simulink model "FormulaElectric"  (R2015a)
settings: Solver=ode1  StartTime=0.0  StopTime=inf  FixedStep=0.001  RelTol=1e-3
InitFcn:
  | %init_dyn_platform
  | FEParameters
StartFcn:
  | tic
StopFcn:
  | toc
undefined symbols (not defined in the file): Battery, Env, magnitude, Motor, RPM2Rad
libraries: vehicleLib x22, mblibv1 x15, driveline x12, fl_lib x8, simulink x6, AMKMotor x4, nesl_utility x4, WheelAssembly x4, ephysenetlib x2, ControllerLib x1, simulink_extras x1
(part 1 of 4)
settings Model: SimulationMode=accelerator  CovSFcnEnable=off  ExtModeTrigDuration=100  Creator=Administrator  LastModifiedBy=tbria
settings SolverCC: ExtrapolationOrder=1
settings DataIOCC: LimitDataPoints=off  MaxDataPoints=1e6  SaveFinalState=on  SaveFormat=StructureWithTime  SaveOutput=off  SaveState=on  SignalLogging=off  StateSaveName=tmp_raccel_xout  SignalLoggingName=tmp_raccel_logsout
settings OptimizationCC: ExpressionDepthLimit=2147483647  InitFltsAndDblsToZero=on  EfficientMapNaN2IntZero=off  SimCompilerOptimization=on
settings DebuggingCC: UnderspecifiedInitializationDetection=Classic  MergeDetectMultiDrivingBlocksExec=none  SolverPrmCheckMsg=warning  InheritedTsInSrcMsg=none  MultiTaskDSMMsg=warning  MultiTaskCondExecSysMsg=none  Int32ToFloatConvMsg=none  ParameterPrecisionLossMsg=none  FcnCallInpInsideContextMsg=EnableAllAsWarning  StateNameClashWarn=warning
settings HardwareCC: ProdHWDeviceType=Generic->32-bit Real-Time Simulator  TargetLongLongMode=on  TargetIntDivRoundTo=Zero  TargetEndianess=LittleEndian  TargetHWDeviceType=MATLAB Host  ProdEqTarget=off
settings CodeAppCC: MaxIdLength=128
settings GRTTargetCC: CombineOutputUpdateFcns=off  GRTInterface=on
settings SimscapeCC: SelectedTab=Simscape

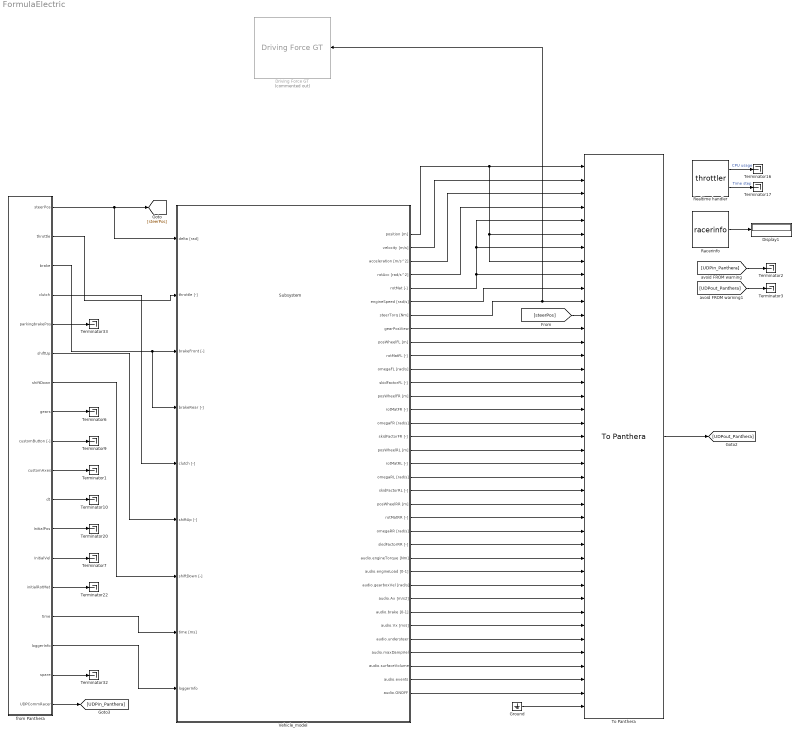
== system FormulaElectric ==
  Display1 : Display
  Driving Force GT : ControllerLib/Driving Force GT  Commented=on
  Ground : Ground
  Racerinfo : S-Function  Priority=5  FunctionName=racerinfo  Parameters=3
  Realtime handler : S-Function  FunctionName=throttler  Parameters=1
  Subsystem : Subsystem
      mask Display: image(imread('crudenlogo_small.jpg','jpg'))
  Terminator{1..3,6..7,9..10,16..17,20,22,32..33} (13 alike) : Terminator
  To Panthera : ephysenetlib/Output blocks/To Panthera
  Vehicle_model : Subsystem
  from Panthera : Subsystem
  wires:
  Vehicle_model/11(omegaFL [rad/s]) -> To Panthera/16
  Vehicle_model/13(posWheelFR [m]) -> To Panthera/18
  Vehicle_model/23(omegaRR [rad/s]) -> To Panthera/28
  To Panthera/1 -> [UDPout_Panthera]
  Vehicle_model/2(velocity [m/s]) -> To Panthera/2
  Vehicle_model/3(acceleration [m/s^2]) -> To Panthera/3
  Vehicle_model/8(gearPosView) -> To Panthera/13
  Vehicle_model/10(rotMatFL [-]) -> To Panthera/15
  Vehicle_model/14(rotMatFR [-]) -> To Panthera/19
  Vehicle_model/12(skidFactorFL [-]) -> To Panthera/17
  Vehicle_model/16(skidFactorFR [-]) -> To Panthera/21
  Vehicle_model/21(posWheelRR [m]) -> To Panthera/26
  Vehicle_model/18(rotMatRL [-]) -> To Panthera/23
  Vehicle_model/22(rotMatRR [-]) -> To Panthera/27
  Vehicle_model/19(omegaRL [rad/s]) -> To Panthera/24
  Vehicle_model/20(skidFactorRL [-]) -> To Panthera/25
  Vehicle_model/24(skidFactorRR [-]) -> To Panthera/29
  Vehicle_model/4(rotAcc [rad/s^2]) -> To Panthera/4
  Vehicle_model/15(omegaFR [rad/s]) -> To Panthera/20
  [steerPos] -> To Panthera/12
  Vehicle_model/17(posWheelRL [m]) -> To Panthera/22
  Racerinfo/1 -> Display1/1
  from Panthera/5(parkingbrakePos) -> Terminator33/1
  from Panthera/8(gears) -> Terminator6/1
  from Panthera/9(customButton [-]) -> Terminator9/1
  from Panthera/11(dt) -> Terminator10/1
  from Panthera/12(InitialPos) -> Terminator20/1
  from Panthera/13(InitialVel) -> Terminator7/1
  from Panthera/14(initialRotMat) -> Terminator22/1
  from Panthera/15(time) -> Vehicle_model/8(time [ms])
  from Panthera/16(loggerInfo) -> Vehicle_model/9(loggerInfo)
  from Panthera/17(spare) -> Terminator32/1
  from Panthera/18(UDPCommRacer) -> [UDPin_Panthera]
  from Panthera/6(shiftUp) -> Vehicle_model/6(shiftUp [-])
  from Panthera/4(clutch) -> Vehicle_model/5(clutch [-])
  Vehicle_model/5(rotMat [-]) -> To Panthera/5, To Panthera/7, To Panthera/9
  Realtime handler/1 -> Terminator16/1  "CPU usage"
  Realtime handler/2 -> Terminator17/1  "Time step"
  Vehicle_model/9(posWheelFL [m]) -> To Panthera/14
  Vehicle_model/25(audio.engineTorque [Nm]) -> To Panthera/30
  Vehicle_model/26(audio.engineLoad [0-1]) -> To Panthera/31
  Vehicle_model/27(audio.gearboxVel [rad/s]) -> To Panthera/32
  Vehicle_model/28(audio.Ax [m/s2]) -> To Panthera/33
  Vehicle_model/29(audio.brake [0-1]) -> To Panthera/34
  Vehicle_model/30(audio.Vx [m/s]) -> To Panthera/35
  Vehicle_model/31(audio.understeer) -> To Panthera/36
  Vehicle_model/32(audio.maxDampVel) -> To Panthera/37
  Vehicle_model/33(audio.surfaceVolume) -> To Panthera/38
  Vehicle_model/34(audio.events) -> To Panthera/39
  Vehicle_model/35(audio.ONOFF) -> To Panthera/40
  Ground/1 -> To Panthera/41
  from Panthera/7(shiftDown) -> Vehicle_model/7(shiftDown [-])
  from Panthera/10(customAxes) -> Terminator1/1
  Vehicle_model/1(position [m]) -> To Panthera/8, To Panthera/6, To Panthera/1
  [UDPout_Panthera] -> Terminator3/1
  [UDPin_Panthera] -> Terminator2/1
  Vehicle_model/6(engineSpeed [rad/s]) -> To Panthera/10
  Vehicle_model/7(steerTorq [Nm]) -> Driving Force GT/1, To Panthera/11
  from Panthera/2(throttle) -> Vehicle_model/2(throttle [-])
  from Panthera/3(brake) -> Vehicle_model/4(brakeRear [-]), Vehicle_model/3(brakeFront [-])
  from Panthera/1(steerPos) -> [steerPos], Vehicle_model/1(delta [rad])

== system FormulaElectric/Subsystem ==

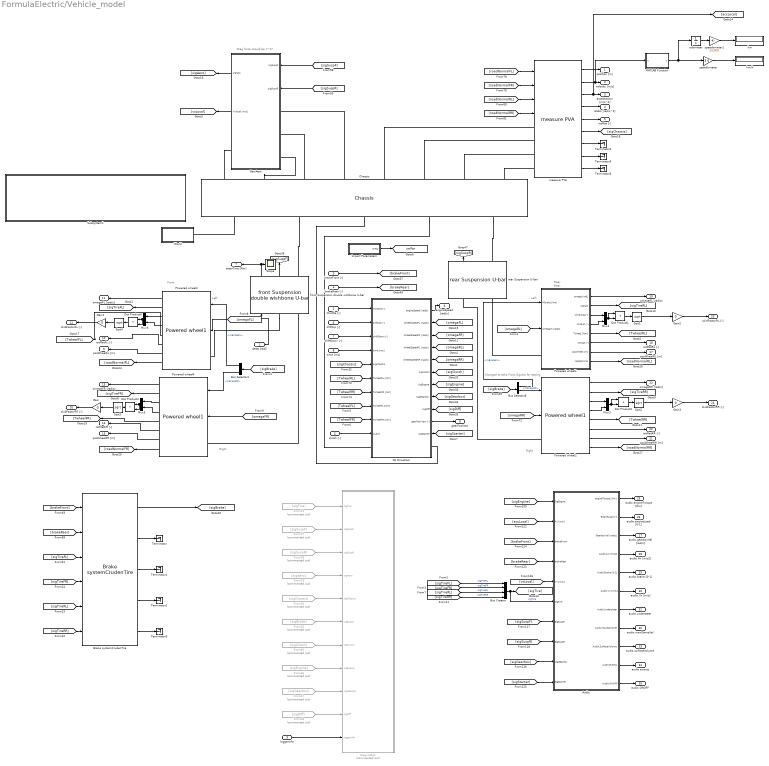
== system FormulaElectric/Vehicle_model ==
  note: Drag force should be V^2?
  note: Changed to take Front Signals for testing
  note: Front
  note: Rear
  note: Left
  note: Right
  note: Right
  note: Left
  note: Rear
  delta [rad] : Inport
  throttle [-] : Inport  Port=2
  brakeFront [-] : Inport  Port=3
  brakeRear [-] : Inport  Port=4
  clutch [-] : Inport  Port=5
  shiftUp [-] : Inport  Port=6
  shiftDown [-] : Inport  Port=7
  time [ms] : Inport  Port=8
  loggerInfo : Inport  Port=9
  Audio : Subsystem
  Brake systemCrudenTire : vehicleLib/Brake system/Total brake system/Brake systemCrudenTire
  Bus Creator : BusCreator
  Bus Selector1 : BusSelector  OutputSignals=mBrakeFL,mBrakeFR
  Bus Selector8 : BusSelector  OutputSignals=mBrakeFL,mBrakeFR
  Chassis : vehicleLib/Chassis/Chassis  massChassis=Veh.Mass  inertiaChassis=[150 0 0; 0 250 0; 0 0 300]  cg=[0.06 0.0 0.3085]  sen=[0.0 0.0 0.3085]  suspFx=0.86  suspRx=-0.765  axleFz=0.338  axleRz=0.3535  posDiff=[-1.16 0.0 0.3085]  posEngine=[0.0 0.0 0.3085]  posFuelTank=[0.0 0.0 0.3085]  cop=[0.0 0.0 0.0]  driverPos=[0.0 0.0 0.3085]  ballastPos=[0.0 0.0 0.3085]  plate0=[0 0 0]  plate1=[0 0 0]  plate2=[0 0 0]  plate3=[0 0 0]  plate4=[0 0 0]  plate5=[0 0 0]  plate6=[0 0 0]  plate7=[0 0 0]
  Diagnostics : Subsystem  Commented=on  mask(Diagnostics){}
      mask help:
      | Diagnostics model collects all the relevant signals from the vehicle model. This model contains among others a logger which outputs its signals to Racer Pro. Racer Pro will produce eg a .rtd log file.
      |
      | Diagnostics model version: V1.0
      |
      | © Cruden B.V., 2012
  Dot Product{1..4} (4 alike) : DotProduct  InputSameDT=on  OutDataTypeStr=Inherit: Inherit via internal rule
  FE Drivetrain : Subsystem  Tag=Power and drivetrain: total power and drivetrain system (do not change this tag)  AncestorBlock=vehicleLib/Power and drivetrain/Complete system/Power and Drivetrain  mask(Power and drivetrain){}
      mask help:
      | Power and drivetrain model based on a conventional power and drivetrain containing an engine, clutch, gearbox and differential. To be used in combination with the SimMechanics multibody and SimDriveline toolbox.
      |
      | Parameters in this model are only used for initialisation during the build process. During simulation with Racer Pro parameters are taken from the car.ini and/or relevant setup.ini.
      |
      | Power and drivetrain model version: V1.0
      |
      | © Cruden B.V., 2012
  From13 : From  Commented=on  GotoTag=sigTire
      settings: CloseFcn=tagdialog Close
  From17 : From  Commented=on  GotoTag=sigSuspF
      settings: CloseFcn=tagdialog Close
  From18 : From  Commented=on  GotoTag=sigSuspR
      settings: CloseFcn=tagdialog Close
  From19 : From  Commented=on  GotoTag=sigAero
      settings: CloseFcn=tagdialog Close
  From20 : From  Commented=on  GotoTag=sigChassis
      settings: CloseFcn=tagdialog Close
  From26 : From  Commented=on  GotoTag=sigBrake
      settings: CloseFcn=tagdialog Close
  From45 : From  Commented=on  GotoTag=sigClutch
      settings: CloseFcn=tagdialog Close
  From46 : From  Commented=on  GotoTag=sigEngine
      settings: CloseFcn=tagdialog Close
  From47 : From  Commented=on  GotoTag=sigGearbox
      settings: CloseFcn=tagdialog Close
  From48 : From  Commented=on  GotoTag=sigDiff
      settings: CloseFcn=tagdialog Close
  Gain{,1..3} (4 alike) : Gain  Gain=0
  Import Parameters : Subsystem
  MATLAB Function : MATLAB Function  TreatAsAtomicUnit=on
  Mux{3..6} (4 alike) : Mux  Inputs=2
  NewAero : Subsystem  Tag=Aerodynamics total system (do not change this tag)  AncestorBlock=vehicleLib/Aerodynamics/Total Aero system/NewAero  mask(Aerodynamics){}
      mask help:
      | Aero model based on measured mappings. To be used in combination with the SimMechanics multibody toolbox.
      |
      | Parameters in this model are only used for initialisation during the build process. During simulation with Racer Pro parameters are taken from the car.ini and/or relevant setup.ini.
      |
      | Aero model version: V1.0
      |
      | © Cruden B.V., 2012
  Powered wheel1 : Subsystem  Tag=Tire and rim: powered wheel (do not change this tag)  AncestorBlock=vehicleLib/Tire and rim/Complete systems/Powered wheel1  mask(Powered wheel){tireNb=2, wheelMass=10, inertiaWheel=diag([0.36 0.48 0.36]), suspX=-0.765, tw=0.7, ahz=0.3535}
      mask prompts: tireNb "Tire number (0-3) [-]"; wheelMass "Wheel mass [kg]"; inertiaWheel "Wheel inertia tensor chassis [3x3] [kgm^2]. The tensor must be a 3-by-3 real, symmetric matrix"; suspX "Distance between Center of Gravity (CG) and center of axle [m]"; tw "Half track width [m]"; ahz "Axle height [m]"
      mask help:
      | Powered wheel model including among others the tire force and moment calculations based on the Magic Formula 6.1. To be used in combination with the SimMechanics multibody toolbox. This is a driven (powered) wheel
      |
      | Parameters in this model are only used for initialisation during the build process. During simulation with Racer Pro parameters are taken from the car.ini and/or relevant setup.ini.
      |
      | Powered wheel model version: V1.0
      |
      | © Cruden B.V., 2012
      mask init:
      | if(tireNb==1 || tireNb==3)
      |   tw=-tw;
      | end
  Powered wheel2 : vehicleLib/Tire and rim/Complete systems/Powered wheel1  Tag=Tire and rim: powered wheel (do not change this tag)  tireNb=3  wheelMass=10  inertiaWheel=diag([0.36 0.48 0.36])  suspX=-0.765  tw=0.7  ahz=0.3535
  Powered wheel3 : vehicleLib/Tire and rim/Complete systems/Powered wheel1  Tag=Tire and rim: powered wheel (do not change this tag)  tireNb=0  wheelMass=10  inertiaWheel=diag([0.36 0.48 0.36])  suspX=0.86  tw=0.654  ahz=0.338
  Powered wheel4 : vehicleLib/Tire and rim/Complete systems/Powered wheel1  Tag=Tire and rim: powered wheel (do not change this tag)  tireNb=1  wheelMass=10  inertiaWheel=diag([0.36 0.48 0.36])  suspX=0.86  tw=0.654  ahz=0.338
  Scope : Scope
      settings: YMin=-2.5  YMax=4  SaveName=ScopeData15
  Sqrt{1..4} (4 alike) : Sqrt  SaturateOnIntegerOverflow=on
  Subsystem1 : Subsystem
      mask Display: image(imread('crudenlogo_medium.jpg','jpg'))
  Terminator{,1..6} (7 alike) : Terminator
  World : Subsystem  mask(World){gravityVector=[0 0 -9.81]}
      mask prompts: gravityVector "Gravity vector [x y z] [m/s^2]"
      mask help:
      | World model represents a six degree of freedom joint which connects the chassis to the SimMechanics environment. To be used in combination with the SimMechanics multibody toolbox.
      |
      | Parameters in this model are used for initialisation during the build process. They are fixed after compilation.
      |
      | World model version: V1.0
      |
      | © Cruden B.V., 2012
  front Suspension double wishbone U-bar : vehicleLib/Suspensions/Complete systems/front Suspension double wishbone U-bar  WFx=0.86  TWF=2*0.654  AHF=0.338  camberFL=-3  camberFR=-3  uprightMass=10  uprightInertia=diag([0.1 0.15 0.9])  massSteerrack=1.8  inertiaSteerrack=diag([0.07 0.1 0.07])  massTorsionbar=1  inertiaTorsionbar=0.1*eye(3)  massRocker=0.6  inertiaRocker=eye(3)  initRHAV=[1.375 0 0.060]  P1="[122.0  116  60]"  P2="[-424  208  112]"  P7="[13  640  73]"  P11="[-20  620  150]"  P3="[110.0  289  297]"  P4="[-434.0  283  246]"  P6="[-80  590  320]"  P5="[176  258  304]"  P8="[78 647  351]"  P12="[-20  296  410]"  P13="[-20  250  380]"  P16="[180 250  380]"  P14="[-26  250  430]"  P21="[-26  300  380]"  P15="[-26  10  430]"  P17="[230  0 100]"  P19="[230  200  100]"  P20="[-26  280  100]"  Z="[247  0.0  280]"  Y="[100  0  289]"  P22="[-20  620  150]"
  km : Display
  km/h : Display
  measure PVA : vehicleLib/Measurement/Total measurement system/measure PVA
  odometer : Integrator
  rear Suspension U-bar : vehicleLib/Suspensions/Complete systems/rear Suspension U-bar  WRx=-0.765  TWR=2*0.7  AHR=0.3535  camberRL=-1  camberRR=-1  uprightMass=10  uprightInertia=diag([0.1 0.15 0.9])  massTorsionbarR=10  massRockerRL=0.6  initRHAR=[0.765 0 0.080]  P1=[278 216 248]  P2="[-240   172  159]"  P7="[51    654  181]"  P11="[28   618  80]"  P3="[280  210 365]"  P4=[-205 190 386]  P6=[10 610 360]  P5="[-240 172  256]"  P8="[-160  618  230]"  P12="[115  160  390]"  P16=[80 145 370]  P13=[80 140 360]  P14=[103 50 450]  P21="[85  108   420]"  P15="[-207  60   450]"  P17="[-367  0.0   215]"  P19=[-367 100.0 215]  P20="[-330   176   450]"  P22="[51    654  181]"  Z1=[-330 0.0 450]  Y1="[-129    0   435]"
  speedometer : Gain  Gain=3.6
  speedometer1 : Gain  Gain=1/1000
  position [m] : Outport
  velocity [m/s] : Outport  Port=2
  acceleration [m/s^2] : Outport  Port=3
  rotAcc [rad/s^2] : Outport  Port=4
  rotMat [-] : Outport  Port=5
  engineSpeed [rad/s] : Outport  Port=6
  steerTorq [Nm] : Outport  Port=7
  gearPosView : Outport  Port=8
  posWheelFL [m] : Outport  Port=9
  rotMatFL [-] : Outport  Port=10
  omegaFL [rad/s] : Outport  Port=11
  skidFactorFL [-] : Outport  Port=12
  posWheelFR [m] : Outport  Port=13
  rotMatFR [-] : Outport  Port=14
  omegaFR [rad/s] : Outport  Port=15
  skidFactorFR [-] : Outport  Port=16
  posWheelRL [m] : Outport  Port=17
  rotMatRL [-] : Outport  Port=18
  omegaRL [rad/s] : Outport  Port=19
  skidFactorRL [-] : Outport  Port=20
  posWheelRR [m] : Outport  Port=21
  rotMatRR [-] : Outport  Port=22
  omegaRR [rad/s] : Outport  Port=23
  skidFactorRR [-] : Outport  Port=24
  audio.engineTorque [Nm] : Outport  Port=25
  audio.engineLoad [0-1] : Outport  Port=26
  audio.gearboxVel [rad/s] : Outport  Port=27
  audio.Ax [m/s2] : Outport  Port=28
  audio.brake [0-1] : Outport  Port=29
  audio.Vx [m/s] : Outport  Port=30
  audio.understeer : Outport  Port=31
  audio.maxDampVel : Outport  Port=32
  audio.surfaceVolume : Outport  Port=33  OutDataTypeStr=double
  audio.events : Outport  Port=34
  audio.ONOFF : Outport  Port=35
  tag scope: imPar=global
  wires:
  shiftDown [-]/1 -> FE Drivetrain/3(shiftDown [-])
  FE Drivetrain/1(engineSpeed [rad/s]) -> engineSpeed [rad/s]/1
  delta [rad]/1 -> front Suspension double wishbone U-bar/1
  NewAero/1(signals) -> [sigAero]
  [sigTireFL] -> Brake systemCrudenTire/3
  [sigTireFR] -> Brake systemCrudenTire/4
  [sigTireRL] -> Brake systemCrudenTire/5
  [sigTireRR] -> Brake systemCrudenTire/6
  time [ms]/1 -> FE Drivetrain/4(time [ms])
  shiftUp [-]/1 -> FE Drivetrain/2(shiftUp [-])
  FE Drivetrain/6(sigClutch) -> [sigClutch]
  FE Drivetrain/7(sigEngine) -> [sigEngine]
  FE Drivetrain/8(sigGearbox) -> [sigGearbox]
  FE Drivetrain/9(sigDiff) -> [sigDiff]
  brakeFront [-]/1 -> [brakeFront]
  [brakeFront] -> Brake systemCrudenTire/1
  brakeRear [-]/1 -> [brakeRear]
  [brakeRear] -> Brake systemCrudenTire/2
  Powered wheel4/1 -> omegaFR [rad/s]/1
  front Suspension double wishbone U-bar/2 -> [sigSuspF]
  rear Suspension U-bar/1 -> [sigSuspR]
  Powered wheel3/1 -> omegaFL [rad/s]/1
  Bus Selector1/1 -> Powered wheel3/1  "<mBrakeFL>"
  [sigBrake] -> Bus Selector1/1
  [sigBrake] -> Bus Selector8/1
  Bus Selector8/2 -> Powered wheel2/1  "<mBrakeFR>"
  Brake systemCrudenTire/1 -> [sigBrake]
  [sigChassis] -> FE Drivetrain/5(sigChassis)
  [TwheelRL] -> FE Drivetrain/6(TwheelRL [Nm])
  [TwheelRR] -> FE Drivetrain/7(TwheelRR [Nm])
  [sigSuspF] -> NewAero/1(sigSuspF)
  [sigSuspR] -> NewAero/2(sigSuspR)
  Powered wheel3/8 -> [roadNormalFL]
  Powered wheel4/8 -> [roadNormalFR]
  [roadNormalFL] -> measure PVA/1
  [roadNormalFR] -> measure PVA/2
  [roadNormalRL] -> measure PVA/3
  [roadNormalRR] -> measure PVA/4
  measure PVA/1 -> position [m]/1
  measure PVA/2 -> MATLAB Function/1(u), velocity [m/s]/1
  measure PVA/4 -> rotAcc [rad/s^2]/1
  measure PVA/5 -> rotMat [-]/1
  measure PVA/6 -> [sigChassis]
  Powered wheel1/7(posWheel [m]) -> posWheelRL [m]/1
  Powered wheel1/6(rotMat [-]) -> rotMatRL [-]/1
  Powered wheel1/5(Twheel [Nm]) -> [TwheelRL]
  Powered wheel1/8(roadNormal) -> [roadNormalRL]
  Powered wheel2/5 -> [TwheelRR]
  Powered wheel2/6 -> rotMatRR [-]/1
  Powered wheel2/7 -> posWheelRR [m]/1
  Powered wheel2/8 -> [roadNormalRR]
  Powered wheel2/2 -> [sigTireRR]
  FE Drivetrain/5(WheelSpeedRR [rad/s]) -> [omegaRR]
  FE Drivetrain/4(WheelSpeedRL [rad/s]) -> [omegaRL]
  [omegaRL] -> Powered wheel1/2(omegaIn [rad/s])
  [omegaRR] -> Powered wheel2/2
  Powered wheel2/1 -> omegaRR [rad/s]/1
  Powered wheel1/1(omega [rad]) -> omegaRL [rad/s]/1
  clutch [-]/1 -> FE Drivetrain/10(clutch)
  throttle [-]/1 -> FE Drivetrain/1(throttle [-])
  Brake systemCrudenTire/5 -> Terminator3/1
  Brake systemCrudenTire/4 -> Terminator2/1
  Brake systemCrudenTire/3 -> Terminator1/1
  Brake systemCrudenTire/2 -> Terminator/1
  [sigSuspF] -> Audio/7(SigSuspF)
  [sigSuspR] -> Audio/8(SigSuspR)
  [brakeRear] -> Audio/4(brakeRear)
  [brakeFront] -> Audio/3(brakeFront)
  [sigEngine] -> Audio/1(SigEngine)
  [vxLocal] -> Audio/5(Vx [m/s])
  [accLocal] -> Audio/2(Ax [m/s])
  [sigGearbox] -> Audio/9(sigGearbox)
  [sigStarter] -> Audio/10(SigStarter)
  Audio/1(engineTorque [Nm]) -> audio.engineTorque [Nm]/1
  Audio/2(EngineLoad [-]) -> audio.engineLoad [0-1]/1
  Audio/3(GearboxVel [rad/s]) -> audio.gearboxVel [rad/s]/1
  Audio/4(Audio.Ax [m/s2]) -> audio.Ax [m/s2]/1
  Audio/5(Audio.Brake [0-1]) -> audio.brake [0-1]/1
  Audio/6(Audio.Vx [m/s]) -> audio.Vx [m/s]/1
  Audio/7(Audio.Understeer) -> audio.understeer/1
  Audio/8(Audio.MaxDampVel) -> audio.maxDampVel/1
  Audio/9(Audio.SurfaceVolume) -> audio.surfaceVolume/1
  Audio/10(Audio.Events) -> audio.events/1
  Audio/11(Audio.ONOFF) -> audio.ONOFF/1
  Bus Creator/1 -> [sigTire], Audio/6(sigTire)  "sigTire"
  [sigTireFL] -> Bus Creator/1  "sigTireFL"
  [sigTireRR] -> Bus Creator/4  "sigTireRR"
  [sigTireFR] -> Bus Creator/2  "sigTireFR"
  [sigTireRL] -> Bus Creator/3  "sigTireRL"
  NewAero/2(Vxlocal [m/s]) -> [vxLocal]
  FE Drivetrain/11(sigStarter) -> [sigStarter]
  Powered wheel3/6 -> rotMatFL [-]/1
  Powered wheel1/2(signals) -> [sigTireRL]
  Dot Product2/1 -> Sqrt2/1
  Sqrt2/1 -> Gain3/1
  Mux3/1 -> Dot Product2/1, Dot Product2/2
  Powered wheel2/4 -> Mux3/2
  Dot Product1/1 -> Sqrt1/1
  Sqrt1/1 -> Gain2/1
  Mux4/1 -> Dot Product1/1, Dot Product1/2
  Powered wheel1/4(skidLat [-]) -> Mux4/2
  Powered wheel1/3(skidLong [-]) -> Mux4/1
  Powered wheel2/3 -> Mux3/1
  Dot Product3/1 -> Sqrt3/1
  Mux5/1 -> Dot Product3/2, Dot Product3/1
  Powered wheel4/3 -> Mux5/1
  Powered wheel4/4 -> Mux5/2
  Dot Product4/1 -> Sqrt4/1
  Mux6/1 -> Dot Product4/2, Dot Product4/1
  Powered wheel3/3 -> Mux6/1
  Sqrt3/1 -> Gain/1
  Sqrt4/1 -> Gain1/1
  measure PVA/7 -> Terminator4/1
  measure PVA/8 -> Terminator5/1
  measure PVA/9 -> Terminator6/1
  measure PVA/3 -> [accLocal], acceleration [m/s^2]/1
  Bus Selector8/1 -> Powered wheel1/1(Mbrake [Nm])  "<mBrakeFL>"
  Import Parameters/1(imPar) -> [imPar]
  From13/1 -> Diagnostics/1(sigTire)
  From19/1 -> Diagnostics/4(sigAero)
  From20/1 -> Diagnostics/5(sigChassis)
  From26/1 -> Diagnostics/6(sigBrake)
  From45/1 -> Diagnostics/7(sigClutch)
  From46/1 -> Diagnostics/8(sigEngine)
  From47/1 -> Diagnostics/9(sigGearbox)
  From48/1 -> Diagnostics/10(sigDiff)
  From17/1 -> Diagnostics/2(sigSuspF)
  From18/1 -> Diagnostics/3(sigSuspR)
  loggerInfo/1 -> Diagnostics/11(loggerInfo)
  FE Drivetrain/3(WheelSpeedFR [rad/s]) -> [omegaFR]
  FE Drivetrain/2(WheelSpeedFL [rad/s]) -> [omegaFL]
  Powered wheel3/4 -> Mux6/2
  Powered wheel4/2 -> [sigTireFR]
  Powered wheel4/6 -> rotMatFR [-]/1
  [TwheelFL] -> FE Drivetrain/8(TwheelFL [Nm])
  [TwheelFR] -> FE Drivetrain/9(TwheelFR [Nm])
  Powered wheel3/2 -> [sigTireFL]
  Powered wheel4/7 -> posWheelFR [m]/1
  Powered wheel3/7 -> posWheelFL [m]/1
  Powered wheel3/5 -> [TwheelFL]
  Powered wheel4/5 -> [TwheelFR]
  [omegaFL] -> Powered wheel3/2
  [omegaFR] -> Powered wheel4/2
  Bus Selector1/2 -> Powered wheel4/1  "<mBrakeFR>"
  Gain/1 -> skidFactorFR [-]/1
  Gain1/1 -> skidFactorFL [-]/1
  Gain2/1 -> skidFactorRL [-]/1
  Gain3/1 -> skidFactorRR [-]/1
  FE Drivetrain/10(gearPosView [-]) -> gearPosView/1
  front Suspension double wishbone U-bar/1 -> Scope/1, steerTorq [Nm]/1
  MATLAB Function/1(y) -> odometer/1, speedometer/1
  speedometer/1 -> km/h/1
  odometer/1 -> speedometer1/1
  speedometer1/1 -> km/1
  connections:
  front Suspension double wishbone U-bar/LConn1 -- Powered wheel3/LConn1
  Powered wheel2/LConn1 -- rear Suspension U-bar/LConn1
  Chassis/LConn1 -- NewAero/RConn1
  Chassis/LConn2 -- NewAero/LConn3
  Chassis/RConn1 -- World/LConn1
  Chassis/RConn2 -- front Suspension double wishbone U-bar/RConn1
  Chassis/RConn4 -- FE Drivetrain/LConn1
  Chassis/LConn3 -- NewAero/LConn2
  Chassis/LConn4 -- NewAero/LConn1
  Chassis/LConn5 -- measure PVA/LConn1
  Chassis/LConn8 -- measure PVA/LConn4
  Chassis/LConn7 -- measure PVA/LConn3
  Chassis/LConn6 -- measure PVA/LConn2
  Chassis/RConn3 -- FE Drivetrain/RConn1
  Powered wheel1/LConn1 -- rear Suspension U-bar/LConn2
  Chassis/RConn5 -- rear Suspension U-bar/RConn1
  front Suspension double wishbone U-bar/LConn2 -- Powered wheel4/LConn1

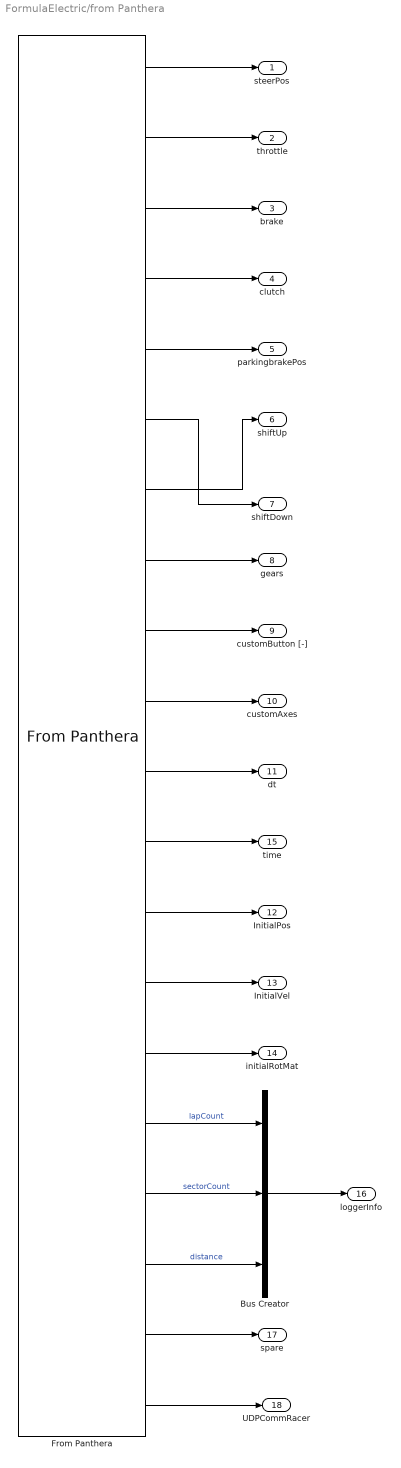
== system FormulaElectric/from Panthera ==
  Bus Creator : BusCreator  Inputs=3
  From Panthera : ephysenetlib/Input blocks/From Panthera
  steerPos : Outport
  throttle : Outport  Port=2
  brake : Outport  Port=3
  clutch : Outport  Port=4
  parkingbrakePos : Outport  Port=5
  shiftUp : Outport  Port=6
  shiftDown : Outport  Port=7
  gears : Outport  Port=8
  customButton [-] : Outport  Port=9
  customAxes : Outport  Port=10
  dt : Outport  Port=11
  InitialPos : Outport  Port=12
  InitialVel : Outport  Port=13
  initialRotMat : Outport  Port=14
  time : Outport  Port=15
  loggerInfo : Outport  Port=16
  spare : Outport  Port=17
  UDPCommRacer : Outport  Port=18
  wires:
  Bus Creator/1 -> loggerInfo/1
  From Panthera/18 -> Bus Creator/3  "distance"
  From Panthera/19 -> spare/1
  From Panthera/13 -> InitialPos/1
  From Panthera/15 -> initialRotMat/1
  From Panthera/12 -> time/1
  From Panthera/14 -> InitialVel/1
  From Panthera/16 -> Bus Creator/1  "lapCount"
  From Panthera/17 -> Bus Creator/2  "sectorCount"
  From Panthera/20 -> UDPCommRacer/1
  From Panthera/1 -> steerPos/1
  From Panthera/10 -> customAxes/1
  From Panthera/2 -> throttle/1
  From Panthera/3 -> brake/1
  From Panthera/7 -> shiftUp/1
  From Panthera/6 -> shiftDown/1
  From Panthera/11 -> dt/1
  From Panthera/9 -> customButton [-]/1
  From Panthera/8 -> gears/1
  From Panthera/5 -> parkingbrakePos/1
  From Panthera/4 -> clutch/1

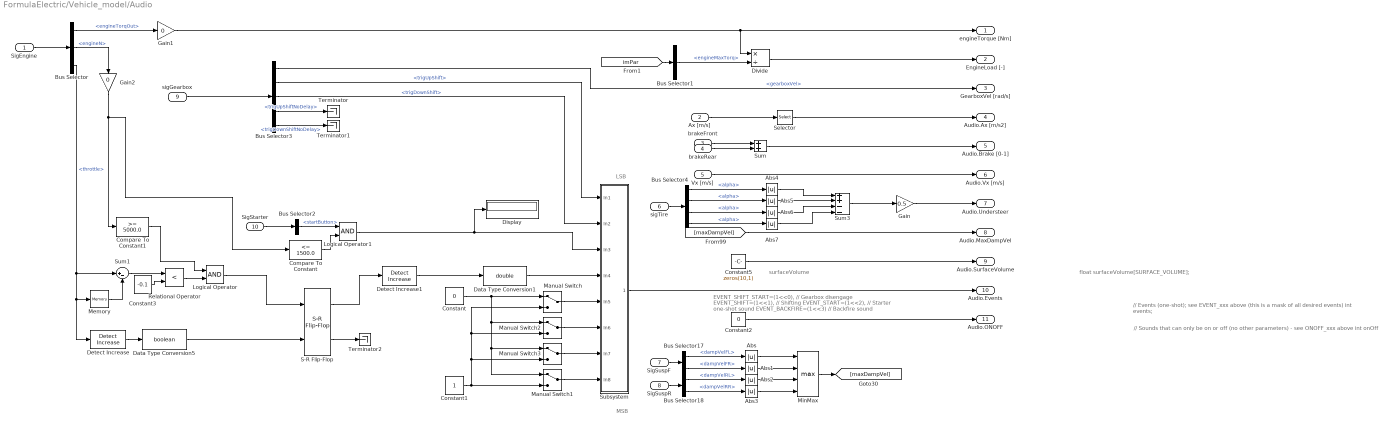
== system FormulaElectric/Vehicle_model/Audio ==
  note: EVENT_SHIFT_START=(1<<0),         // Gearbox disengage
      | EVENT_SHIFT=(1<<1),               // Shifting
      | EVENT_START=(1<<2),               // Starter one-shot sound
      | EVENT_BACKFIRE=(1<<3)             // Backfire sound
  note: MSB
  note: LSB
  note: surfaceVolume
  note: // Sounds that can only be on or off (no other parameters) - see ONOFF_xxx above
      |   int   onOff
  note: // Events (one-shot); see EVENT_xxx above (this is a mask of all desired events)
      |   int   events;
  note: float surfaceVolume[SURFACE_VOLUME];
  SigEngine : Inport
  Ax [m/s] : Inport  Port=2
  brakeFront : Inport  Port=3
  brakeRear : Inport  Port=4
  Vx [m/s] : Inport  Port=5
  sigTire : Inport  Port=6
  SigSuspF : Inport  Port=7
  SigSuspR : Inport  Port=8
  sigGearbox : Inport  Port=9
  SigStarter : Inport  Port=10
  Abs{,1..7} (8 alike) : Abs
  Bus Selector : BusSelector  OutputSignals=engineTorqOut,engineN,throttle
  Bus Selector1 : BusSelector  OutputSignals=engineMaxTorq
  Bus Selector17 : BusSelector  OutputSignals=sigSprDamperL.dampVelFL,sigSprDamperR.dampVelFR
  Bus Selector18 : BusSelector  OutputSignals=sigSprDamperL.dampVelRL,sigSprDamperR.dampVelRR
  Bus Selector2 : BusSelector  OutputSignals=startButton
  Bus Selector3 : BusSelector  OutputSignals=gearboxVel,trigUpShift,trigDownShift,trigUpShiftNoDelay,trigDownShiftNoDelay
  Bus Selector4 : BusSelector  OutputSignals=sigTireFL.alpha,sigTireFR.alpha,sigTireRL.alpha,sigTireRR.alpha
  Compare To Constant : simulink/Logic and Bit Operations/Compare To Constant  relop=<=  const=1500.0  OutDataTypeStr=uint8
  Compare To Constant1 : simulink/Logic and Bit Operations/Compare To Constant  relop=>=  const=5000.0  OutDataTypeStr=uint8
  Constant : Constant  Value=0
  Constant1 : Constant
  Constant2 : Constant  Value=0
  Constant3 : Constant  Value=-0.1
  Constant5 : Constant  Value=zeros(10,1)
  Data Type Conversion1 : DataTypeConversion  OutDataTypeStr=double
  Data Type Conversion5 : DataTypeConversion  OutDataTypeStr=boolean
  Detect Increase : simulink/Logic and Bit Operations/Detect Increase  vinit=0.0  InputProcessing=Inherited  OutDataTypeStr=uint8
  Detect Increase1 : simulink/Logic and Bit Operations/Detect Increase  vinit=0.0  InputProcessing=Inherited  OutDataTypeStr=uint8
  Display : Display
  Divide : Product  Inputs=*/
  Gain : Gain  Gain=0.5
  Gain1 : Gain  Gain=0
  Gain2 : Gain  Gain=0
  Logical Operator : Logic  AllPortsSameDT=off  OutDataTypeStr=boolean
  Logical Operator1 : Logic  AllPortsSameDT=off  OutDataTypeStr=boolean
  Manual Switch{,1..3} (4 alike) : ManualSwitch
  Memory : Memory  InheritSampleTime=on  LinearizeAsDelay=on
  MinMax : MinMax  Function=max  Inputs=4
  Relational Operator : RelationalOperator  Operator=<  OutDataTypeStr=boolean
  S-R Flip-Flop : simulink_extras/Flip Flops/S-R Flip-Flop  initial_condition=0
  Selector : Selector  InputPortWidth=3  Indices=[1]
  Subsystem : Subsystem
  Sum : Sum
  Sum1 : Sum  Inputs=|+-
  Sum3 : Sum  Inputs=++--
  Terminator : Terminator
  Terminator1 : Terminator
  Terminator2 : Terminator
  engineTorque [Nm] : Outport
  EngineLoad [-] : Outport  Port=2
  GearboxVel [rad/s] : Outport  Port=3
  Audio.Ax [m/s2] : Outport  Port=4
  Audio.Brake [0-1] : Outport  Port=5
  Audio.Vx [m/s] : Outport  Port=6
  Audio.Understeer : Outport  Port=7
  Audio.MaxDampVel : Outport  Port=8
  Audio.SurfaceVolume : Outport  Port=9
  Audio.Events : Outport  Port=10
  Audio.ONOFF : Outport  Port=11
  wires:
  Compare To Constant1/1 -> Logical Operator/1
  Logical Operator/1 -> S-R Flip-Flop/1
  Relational Operator/1 -> Logical Operator/2
  Bus Selector/2 -> Gain2/1  "<engineN>"
  Constant3/1 -> Relational Operator/2
  Sum1/1 -> Relational Operator/1
  Memory/1 -> Sum1/2
  Bus Selector3/2 -> Subsystem/1(In1)  "<trigUpShift>"
  Bus Selector3/3 -> Subsystem/2(In2)  "<trigDownShift>"
  Bus Selector3/5 -> Terminator1/1  "<trigDownShiftNoDelay>"
  Bus Selector3/4 -> Terminator/1  "<trigUpShiftNoDelay>"
  sigGearbox/1 -> Bus Selector3/1
  SigStarter/1 -> Bus Selector2/1
  Divide/1 -> EngineLoad [-]/1
  Bus Selector/1 -> Gain1/1  "<engineTorqOut>"
  Bus Selector1/1 -> Divide/2  "<engineMaxTorq>"
  [imPar] -> Bus Selector1/1
  Constant5/1 -> Audio.SurfaceVolume/1
  [maxDampVel] -> Audio.MaxDampVel/1
  Sum3/1 -> Gain/1
  Subsystem/1(Out1) -> Audio.Events/1
  Constant/1 -> Manual Switch3/1, Manual Switch1/1, Manual Switch2/1, Manual Switch/1
  Constant1/1 -> Manual Switch/2, Manual Switch2/2, Manual Switch3/2, Manual Switch1/2
  Manual Switch3/1 -> Subsystem/7(In7)
  Manual Switch2/1 -> Subsystem/6(In6)
  Manual Switch/1 -> Subsystem/5(In5)
  Manual Switch1/1 -> Subsystem/8(In8)
  SigSuspR/1 -> Bus Selector18/1
  SigSuspF/1 -> Bus Selector17/1
  sigTire/1 -> Bus Selector4/1
  brakeRear/1 -> Sum/2
  brakeFront/1 -> Sum/1
  Ax [m/s]/1 -> Selector/1
  Bus Selector3/1 -> GearboxVel [rad/s]/1  "<gearboxVel>"
  SigEngine/1 -> Bus Selector/1
  Vx [m/s]/1 -> Audio.Vx [m/s]/1
  Constant2/1 -> Audio.ONOFF/1
  Selector/1 -> Audio.Ax [m/s2]/1
  Sum/1 -> Audio.Brake [0-1]/1
  MinMax/1 -> [maxDampVel]
  Bus Selector18/2 -> Abs3/1  "<dampVelRR>"
  Bus Selector18/1 -> Abs2/1  "<dampVelRL>"
  Bus Selector17/2 -> Abs1/1  "<dampVelFR>"
  Abs/1 -> MinMax/1
  Abs1/1 -> MinMax/2
  Abs2/1 -> MinMax/3
  Abs3/1 -> MinMax/4
  Bus Selector17/1 -> Abs/1  "<dampVelFL>"
  Bus Selector2/1 -> Logical Operator1/1  "<startButton>"
  Compare To Constant/1 -> Logical Operator1/2
  Logical Operator1/1 -> Subsystem/3(In3), Display/1
  Detect Increase/1 -> Data Type Conversion5/1
  Data Type Conversion5/1 -> S-R Flip-Flop/2
  S-R Flip-Flop/2 -> Terminator2/1
  S-R Flip-Flop/1 -> Detect Increase1/1
  Detect Increase1/1 -> Data Type Conversion1/1
  Data Type Conversion1/1 -> Subsystem/4(In4)
  Bus Selector/3 -> Sum1/1, Memory/1, Detect Increase/1  "<throttle>"
  Bus Selector4/1 -> Abs4/1  "<alpha>"
  Bus Selector4/2 -> Abs5/1  "<alpha>"
  Bus Selector4/3 -> Abs6/1  "<alpha>"
  Bus Selector4/4 -> Abs7/1  "<alpha>"
  Abs4/1 -> Sum3/1
  Abs5/1 -> Sum3/2
  Abs6/1 -> Sum3/3
  Abs7/1 -> Sum3/4
  Gain/1 -> Audio.Understeer/1
  Gain1/1 -> Divide/1, engineTorque [Nm]/1
  Gain2/1 -> Compare To Constant/1, Compare To Constant1/1

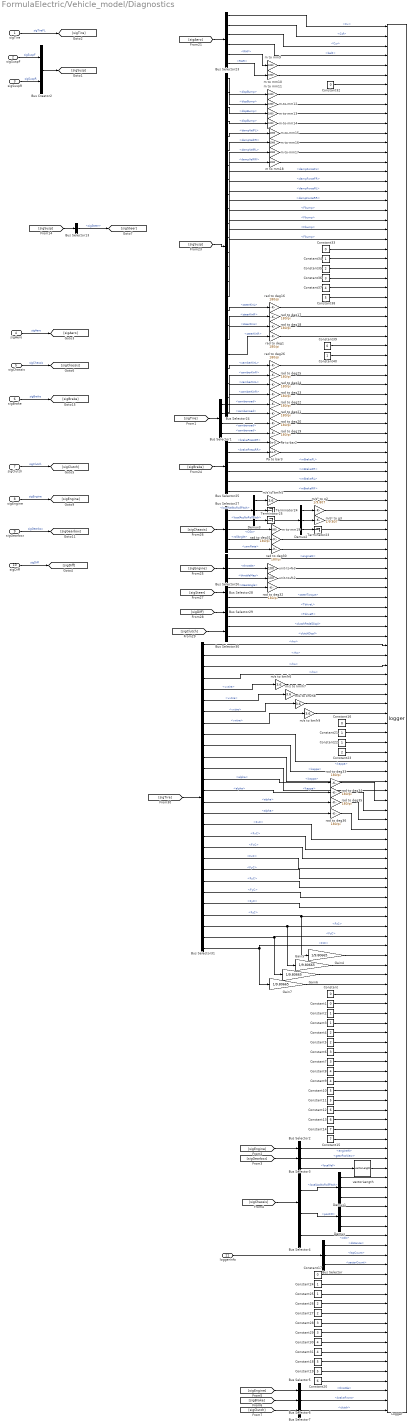
== system FormulaElectric/Vehicle_model/Diagnostics ==
  sigTire : Inport
  sigSuspF : Inport  Port=2
  sigSuspR : Inport  Port=3
  sigAero : Inport  Port=4
  sigChassis : Inport  Port=5
  sigBrake : Inport  Port=6
  sigClutch : Inport  Port=7
  sigEngine : Inport  Port=8
  sigGearbox : Inport  Port=9
  sigDiff : Inport  Port=10
  loggerInfo : Inport  Port=11
  Bus Creator2 : BusCreator  Inputs=2
  Bus Selector : BusSelector  OutputSignals=distance,lapCount,sectorCount
  Bus Selector1 : BusSelector  OutputSignals=sigTireFL.camberroad,sigTireFR.camberroad,sigTireRL.camberroad,sigTireRR.camberroad
  Bus Selector13 : BusSelector  OutputSignals=sigSuspF.sigSteer
  Bus Selector2 : BusSelector  OutputSignals=engineN
  Bus Selector23 : BusSelector  OutputSignals=Cx,Czf,Czr,balF,RHF,RHR
  Bus Selector24 : BusSelector  OutputSignals=sigSuspF.sigSprDamperL.dispBump,sigSuspF.sigSprDamperR.dispBump,sigSuspR.sigSprDamperL.dispBump,sigSuspR.sigSprDamperR.dispBump,sigSuspF.sigSprDamperL.dampVelFL,sigSuspF.sigSprDamperR.dampVelFR,sigSuspR.sigSprDamperL.dampVelRL,sigSuspR.sigSprDamperR.dampVelRR,sigSuspF.sigSprDamperL.dampForceFL,sigSuspF.sigSprDamperR.dampForceFR,sigSuspR.sigSprDamperL.dampForceRL,sigSuspR.sigSprDamperR.dampForceRR,sigSuspF.sigSprDamperL.Fbump,sigSuspF.sigSprDamperR.Fbump,sigSuspR.sigSprDamperL.Fbump,sigSuspR.sigSprDamperR.Fbump,sigSuspF.sigToe.steerKinL,sigSuspF.sigToe.steerKinR,sigSuspR.sigToe.steerKinL,sigSuspR.sigToe.steerKinR,sigSuspF.sigCamber.camberKinL,sigSuspF.sigCamber.camberKinR,sigSuspR.sigCamber.camberKinL,sigSuspR.sigCamber.camberKinR
  Bus Selector25 : BusSelector  OutputSignals=brakePressFR,brakePressRR,mBrakeFL,mBrakeFR,mBrakeRL,mBrakeRR
  Bus Selector26 : BusSelector  OutputSignals=engineN,throttle,throttleMap
  Bus Selector27 : BusSelector  OutputSignals=localVelNoRollPitch,localAccNoRollPitch,CGz,rollAngle,yawRate
  Bus Selector28 : BusSelector  OutputSignals=steerAngle,steerTorque
  Bus Selector29 : BusSelector  OutputSignals=TdriveL,TdriveR
  Bus Selector3 : BusSelector  OutputSignals=gearPosView
  Bus Selector30 : BusSelector  OutputSignals=clutchPedalDispl,clutchDispl
  Bus Selector31 : BusSelector  OutputSignals=sigTireFL.rho,sigTireFR.rho,sigTireRL.rho,sigTireRR.rho,sigTireFL.vxtire,sigTireFR.vxtire,sigTireRL.vxtire,sigTireRR.vxtire,sigTireFL.kappa,sigTireFR.kappa,sigTireRL.kappa,sigTireRR.kappa,sigTireFL.alpha,sigTireFR.alpha,sigTireRL.alpha,sigTireRR.alpha,sigTireFL.FxC,sigTireFR.FxC,sigTireRL.FxC,sigTireRR.FxC,sigTireFL.FyC,sigTireFR.FyC,sigTireRL.FyC,sigTireRR.FyC,sigTireFL.FzC,sigTireFR.FzC,sigTireRL.FzC,sigTireRR.FzC
  Bus Selector4 : BusSelector  OutputSignals=localVel,localAccNoRollPitch,posCG,odo
  Bus Selector5 : BusSelector  OutputSignals=throttle
  Bus Selector6 : BusSelector  OutputSignals=brakeFront
  Bus Selector7 : BusSelector  OutputSignals=clutch
  Constant{,1,16..17,32..33,39} (7 alike) : Constant  Value=0
  Constant{10..11,18..19,38} (5 alike) : Constant  Value=5
  Constant12 : Constant  Value=6
  Constant13 : Constant  Value=6
  Constant14 : Constant  Value=7
  Constant15 : Constant  Value=7
  Constant{2..3,21..22,24..25,34,40} (8 alike) : Constant
  Constant20 : Constant  Value=6
  Constant{4..5,23,26..27,35} (6 alike) : Constant  Value=2
  Constant{6..7,28..29,36} (5 alike) : Constant  Value=3
  Constant{8..9,30..31,37} (5 alike) : Constant  Value=4
  Demux{,1..3} (4 alike) : Demux  Outputs=3
  Gain{4..7} (4 alike) : Gain  Gain=1/9.80665
  Logger : S-Function  FunctionName=logger  Parameters=1
      mask Display:
      | % port_label('input',1,'aero_cx')
      | % port_label('input',2,'aero_czf')
      | % port_label('input',3,'aero_czr')
      | % port_label('input',4,'aero_balance')
      | % port_label('input',5,'e_rh_front')
      | % port_label('input',6,'e_rh_rear')
      | % port_label('input',7,'B_wing_open')
      | % port_label('input',8,'sdam_fl')
      | % port_label('input',9,'sdam_fr')
      | % port_label('input',10,'sdam_rl')
      | % port_label('input',11,'sdam_rr')
      | % port_label('input',12,'vdam_fl')
      | % port_label('input',13,'vdam_fr')
      | % port_label('input',14,'vdam_rl')
      | % port_label('input',15,'vdam_rr')
      | % port_label('input',16,'fdam_fl')
      | % port_label('input',17,'fdam_fr')
      | % port_label('input',18,'fdam_rl')
      | % port_label('input',19,'fdam_rr')
      | % port_label('input',20,'f_bump_fl')
      | % port_label('input',21,'f_bump_fr')
      | % port_label('input',22,'f_bump_rl')
      | % port_label('input',23,'f_bump_rr')
      | % port_label('input',24,'f_arb_front')
      | % port_label('input',25,'f_arb_rear')
      | % port_label('input',26,'e_EFA_front')
      | % port_label('input',27,'f_EFA_front')
      | % port_label('input',28,'e_EFA_rear')
      | % port_label('input',29,'f_EFA_rear')
      | % port_label('input',30,'steer_fl')
      | % port_label('input',31,'steer_fr')
      | % port_label('input',32,'steer_rl')
      | % port_label('input',33,'steer_rr')
      | % port_label('input',34,'castor_fl')
      | % port_label('input',35,'castor_fr')
      | % port_label('input',36,'camber_fl_chassis')
      | % port_label('input',37,'camber_fr_chassis')
      | % port_label('input',38,'camber_rl_chassis')
      | % port_label('input',39,'camber_rr_chassis')
      | % port_label('input',40,'camber_fl_road')
      | % port_label('input',41,'camber_fr_road')
      | % port_label('input',42,'camber_rl_road')
      | % port_label('input',43,'camber_rr_road')
      | % port_label('input',44,'pbrake_f')
      | % port_label('input',45,'pbrake_r')
      | % port_label('input',46,'brake_torque_fl')
      | % port_label('input',47,'brake_torque_fr')
      | % port_label('input',48,'brake_torque_rl')
      | % port_label('input',49,'brake_torque_rr')
      | % port_label('input',50,'speed')
      | % port_label('input',51,'accx_r')
      | % port_label('input',52,'accy_r')
      | % port_label('input',53,'CG_height')
      | % port_label('input',54,'roll_angle')
      | % port_label('input',55,'yaw_rate')
      | % port_label('input',56,'nmot')
      | % port_label('input',57,'aps')
      | % port_label('input',58,'ath')
      | % port_label('input',59,'steer')
      | % port_label('input',60,'steerTorqRAW')
      | % port_label('input',61,'drive_torque_rl')
      | % port_label('input',62,'drive_torque_rr')
      | % port_label('input',63,'clutch_displacement')
      | % port_label('input',64,'pclutch')
      | % port_label('input',65,'tire_deflection_fl')
      | % port_label('input',66,'tire_deflection_fr')
      | % port_label('input',67,'tire_deflection_rl')
      | % port_label('input',68,'tire_deflection_rr')
      | % port_label('input',69,'vwheel_fl')
      | % port_label('input',70,'vwheel_fr')
      | % port_label('input',71,'vwheel_rl')
      | % port_label('input',72,'vwheel_rr')
      | % port_label('input',73,'omega_fl')
      | % port_label('input',74,'omega_fr')
      | % port_label('input',75,'omega_rl')
      | % port_label('input',76,'omega_rr')
      | % port_label('input',77,'slip_ratio_fl')
      | % port_label('input',78,'slip_ratio_fr')
      | % port_label('input',79,'slip_ratio_rl')
      | % port_label('input',80,'slip_ratio_rr')
      | % port_label('input',81,'slip_angle_fl')
      | % port_label('input',82,'slip_angle_fr')
      | % port_label('input',83,'slip_angle_rl')
      | % port_label('input',84,'slip_angle_rr')
      | % port_label('input',85,'tire_Fx_fl')
      | % port_label('input',86,'tire_Fx_fr')
      | % port_label('input',87,'tire_Fx_rl')
      | % port_label('input',88,'tire_Fx_rr')
      | % port_label('input',89,'tire_Fy_fl')
      | % port_label('input',90,'tire_Fy_fr')
      | % port_label('input',91,'tire_Fy_rl')
      | % port_label('input',92,'tire_Fy_rr')
      | % port_label('input',93,'tire_Fz_fl')
      | % port_label('input',94,'tire_Fz_fr')
      | % port_label('input',95,'tire_Fz_rl')
      | % port_label('input',96,'tire_Fz_rr')
      | % port_label('input',97,'dms_fl')
      | % port_label('input',98,'dms_fr')
      | % port_label('input',99,'dms_rl')
      | % port_label('input',100,'dms_rr')
      | % port_label('input',101,'plate0_dist')
      | % port_label('input',102,'plate0_force')
      | % port_label('input',103,'plate1_dist')
      | % port_label('input',104,'plate1_force')
      | % port_label('input',105,'plate2_dist')
      | % port_label('input',106,'plate2_force')
      | % port_label('input',107,'plate3_dist')
      | % port_label('input',108,'plate3_force')
      | % port_label('input',109,'plate4_dist')
      | % port_label('input',110,'plate4_force')
      | % port_label('input',111,'plate5_dist')
      | % port_label('input',112,'plate5_force')
      | % port_label('input',113,'plate6_dist')
      | % port_label('input',114,'plate6_force')
      | % port_label('input',115,'plate7_dist')
      | % port_label('input',116,'plate7_force')
      | % port_label('input',117,'rpm')
      | % port_label('input',118,'gear')
      | % port_label('input',119,'velocity')
      | % port_label('input',120,'acc_x')
      | % port_label('input',121,'acc_y')
      | % port_label('input',122,'acc_z')
      | % port_label('input',123,'pos_x')
      | % port_label('input',124,'pos_y')
      | % port_label('input',125,'pos_z')
      | % port_label('input',126,'odometer')
      | % port_label('input',127,'distance')
      | % port_label('input',128,'lap')
      | % port_label('input',129,'sector')
      | % port_label('input',130,'flags')
      | % port_label('input',131,'custom0')
      | % port_label('input',132,'custom1')
      | % port_label('input',133,'custom2')
      | % port_label('input',134,'custom3')
      | % port_label('input',135,'custom4')
      | % port_label('input',136,'custom5')
      | % port_label('input',137,'custom6')
      | % port_label('input',138,'custom7')
      | % port_label('input',139,'custom8')
      | % port_label('input',140,'custom9')
      | % port_label('input',141,'custom10')
      | % port_label('input',142,'throttle')
      | % port_label('input',143,'brakes')
      | % port_label('input',144,'clutch')
      | %
      | A=fileread('logger_variables.h');
      | p=0;
      | namen=[];
      | %A
      | for k=6:length(A)-5;
      |     if strcmp(A(k-4:k),'    "')
      |         l=0;
      |         isfound=0;
      |         while ~isfound
      |             l=l+1;
      |             isfound=strcmp(A(k+l:k+l+1),'",');
      |         end %while
      |         name=A(k+1:k+l-1);
      |         p=p+1;
      |         port_label('input',p,name)
      |         %port_label('output',p,name)
      |     end %if
      | end %for
  Pa to bar2 : Gain  Gain=1e-5
  Pa to bar3 : Gain  Gain=1e-5
  Terminator23 : Terminator
  Terminator24 : Terminator
  Terminator25 : Terminator
  m to mm{9..19} (11 alike) : Gain  Gain=1000
  m/s to km/h{5..9} (5 alike) : Gain  Gain=3.6
  m/s² to g2 : Gain  Gain=1/9.807
  m/s² to g3 : Gain  Gain=1/9.807
  rad to deg{1,16..26,30..36} (19 alike) : Gain  Gain=180/pi
  unit to %2 : Gain  Gain=100
  unit to %3 : Gain  Gain=100
  vectorLength : vehicleLib/Utilities/vectorLength
  wires:
  Bus Selector13/1 -> [sigSteer]  "<sigSteer>"
  [sigSusp] -> Bus Selector13/1
  Bus Creator2/1 -> [sigSusp]
  sigSuspR/1 -> Bus Creator2/2  "sigSuspR"
  sigSuspF/1 -> Bus Creator2/1  "sigSuspF"
  sigDiff/1 -> [sigDiff]  "sigDiff"
  sigGearbox/1 -> [sigGearbox]  "sigGearbox"
  sigEngine/1 -> [sigEngine]  "sigEngine"
  sigClutch/1 -> [sigClutch]  "sigClutch"
  sigAero/1 -> [sigAero]  "sigAero"
  sigChassis/1 -> [sigChassis]  "sigChassis"
  sigBrake/1 -> [sigBrake]  "sigBrake"
  sigTire/1 -> [sigTire]  "sigTireFL"
  [sigAero] -> Bus Selector23/1
  m to mm10/1 -> Logger/6
  m to mm9/1 -> Logger/5
  Bus Selector23/6 -> m to mm10/1  "<RHR>"
  Bus Selector23/5 -> m to mm9/1  "<RHF>"
  Bus Selector23/4 -> Logger/4  "<balF>"
  Bus Selector23/3 -> Logger/3  "<Czr>"
  Bus Selector23/2 -> Logger/2  "<Czf>"
  Bus Selector23/1 -> Logger/1  "<Cx>"
  [sigSusp] -> Bus Selector24/1
  Bus Selector24/1 -> m to mm11/1  "<dispBump>"
  Bus Selector24/2 -> m to mm12/1  "<dispBump>"
  Bus Selector24/3 -> m to mm13/1  "<dispBump>"
  Bus Selector24/4 -> m to mm14/1  "<dispBump>"
  m to mm11/1 -> Logger/8
  m to mm12/1 -> Logger/9
  m to mm13/1 -> Logger/10
  m to mm14/1 -> Logger/11
  Bus Selector24/5 -> m to mm15/1  "<dampVelFL>"
  Bus Selector24/6 -> m to mm16/1  "<dampVelFR>"
  Bus Selector24/7 -> m to mm17/1  "<dampVelRL>"
  Bus Selector24/8 -> m to mm18/1  "<dampVelRR>"
  Bus Selector24/9 -> Logger/16  "<dampForceFL>"
  Bus Selector24/10 -> Logger/17  "<dampForceFR>"
  Bus Selector24/11 -> Logger/18  "<dampForceRL>"
  Bus Selector24/12 -> Logger/19  "<dampForceRR>"
  Bus Selector24/13 -> Logger/20  "<Fbump>"
  Bus Selector24/14 -> Logger/21  "<Fbump>"
  Bus Selector24/15 -> Logger/22  "<Fbump>"
  Bus Selector24/16 -> Logger/23  "<Fbump>"
  Bus Selector24/17 -> rad to deg16/1  "<steerKinL>"
  Bus Selector24/18 -> rad to deg17/1  "<steerKinR>"
  Bus Selector24/19 -> rad to deg18/1  "<steerKinL>"
  Bus Selector24/20 -> rad to deg1/1  "<steerKinR>"
  rad to deg16/1 -> Logger/30
  rad to deg17/1 -> Logger/31
  rad to deg18/1 -> Logger/32
  Bus Selector24/22 -> rad to deg25/1  "<camberKinR>"
  Bus Selector24/23 -> rad to deg24/1  "<camberKinL>"
  Bus Selector24/24 -> rad to deg23/1  "<camberKinR>"
  Bus Selector24/21 -> rad to deg26/1  "<camberKinL>"
  rad to deg20/1 -> Logger/42
  rad to deg21/1 -> Logger/41
  rad to deg22/1 -> Logger/40
  rad to deg23/1 -> Logger/39
  rad to deg24/1 -> Logger/38
  rad to deg25/1 -> Logger/37
  rad to deg26/1 -> Logger/36
  Constant40/1 -> Logger/35
  Constant39/1 -> Logger/34
  rad to deg1/1 -> Logger/33
  m to mm15/1 -> Logger/12
  m to mm16/1 -> Logger/13
  m to mm17/1 -> Logger/14
  m to mm18/1 -> Logger/15
  rad to deg19/1 -> Logger/43
  [sigBrake] -> Bus Selector25/1
  Bus Selector25/1 -> Pa to bar2/1  "<brakePressFR>"
  Bus Selector25/2 -> Pa to bar3/1  "<brakePressRR>"
  Bus Selector25/3 -> Logger/46  "<mBrakeFL>"
  Bus Selector25/4 -> Logger/47  "<mBrakeFR>"
  Bus Selector25/5 -> Logger/48  "<mBrakeRL>"
  Bus Selector25/6 -> Logger/49  "<mBrakeRR>"
  Pa to bar2/1 -> Logger/44
  Pa to bar3/1 -> Logger/45
  Demux2/3 -> Terminator23/1
  Demux2/2 -> m/s² to g3/1
  Demux2/1 -> m/s² to g2/1
  [sigChassis] -> Bus Selector27/1
  Demux3/2 -> Terminator24/1
  Demux3/3 -> Terminator25/1
  Demux3/1 -> m/s to km/h5/1
  Bus Selector27/1 -> Demux3/1  "<localVelNoRollPitch>"
  Bus Selector27/2 -> Demux2/1  "<localAccNoRollPitch>"
  Bus Selector27/3 -> m to mm19/1  "<CGz>"
  Bus Selector27/5 -> rad to deg30/1  "<yawRate>"
  Bus Selector27/4 -> rad to deg31/1  "<rollAngle>"
  m/s² to g3/1 -> Logger/52
  m/s² to g2/1 -> Logger/51
  m/s to km/h5/1 -> Logger/50
  rad to deg30/1 -> Logger/55
  rad to deg31/1 -> Logger/54
  m to mm19/1 -> Logger/53
  unit to %3/1 -> Logger/57
  Bus Selector26/2 -> unit to %3/1  "<throttle>"
  unit to %2/1 -> Logger/58
  Bus Selector26/1 -> Logger/56  "<engineN>"
  Bus Selector26/3 -> unit to %2/1  "<throttleMap>"
  [sigEngine] -> Bus Selector26/1
  rad to deg32/1 -> Logger/59
  Bus Selector28/1 -> rad to deg32/1  "<steerAngle>"
  [sigSteer] -> Bus Selector28/1
  Bus Selector28/2 -> Logger/60  "<steerTorque>"
  Bus Selector29/2 -> Logger/62  "<TdriveR>"
  Bus Selector29/1 -> Logger/61  "<TdriveL>"
  [sigDiff] -> Bus Selector29/1
  Bus Selector30/2 -> Logger/64  "<clutchDispl>"
  [sigClutch] -> Bus Selector30/1
  [sigTire] -> Bus Selector31/1
  Bus Selector30/1 -> Logger/63  "<clutchPedalDispl>"
  Constant16/1 -> Logger/73
  Constant21/1 -> Logger/74
  Constant22/1 -> Logger/75
  Constant23/1 -> Logger/76
  m/s to km/h6/1 -> Logger/69
  Bus Selector31/5 -> m/s to km/h6/1  "<vxtire>"
  Bus Selector31/8 -> m/s to km/h9/1  "<vxtire>"
  Bus Selector31/7 -> m/s to km/h8/1  "<vxtire>"
  Bus Selector31/6 -> m/s to km/h7/1  "<vxtire>"
  m/s to km/h7/1 -> Logger/70
  m/s to km/h8/1 -> Logger/71
  m/s to km/h9/1 -> Logger/72
  Bus Selector31/21 -> Logger/89  "<FyC>"
  Bus Selector31/22 -> Logger/90  "<FyC>"
  Bus Selector31/23 -> Logger/91  "<FyC>"
  Bus Selector31/24 -> Logger/92  "<FyC>"
  Bus Selector31/25 -> Gain4/1, Logger/93  "<FzC>"
  Bus Selector31/26 -> Gain5/1, Logger/94  "<FzC>"
  Bus Selector31/27 -> Logger/95, Gain6/1  "<FzC>"
  Bus Selector31/28 -> Logger/96, Gain7/1  "<FzC>"
  Gain4/1 -> Logger/97
  Gain5/1 -> Logger/98
  Gain6/1 -> Logger/99
  Gain7/1 -> Logger/100
  rad to deg33/1 -> Logger/81
  rad to deg34/1 -> Logger/82
  rad to deg35/1 -> Logger/83
  rad to deg36/1 -> Logger/84
  [sigTire] -> Bus Selector1/1
  Bus Selector1/1 -> rad to deg22/1  "<camberroad>"
  Bus Selector1/2 -> rad to deg21/1  "<camberroad>"
  Bus Selector1/3 -> rad to deg20/1  "<camberroad>"
  Bus Selector1/4 -> rad to deg19/1  "<camberroad>"
  Constant/1 -> Logger/101
  Constant1/1 -> Logger/102
  Constant2/1 -> Logger/103
  Constant3/1 -> Logger/104
  Constant4/1 -> Logger/105
  Constant5/1 -> Logger/106
  Constant6/1 -> Logger/107
  Constant7/1 -> Logger/108
  Constant8/1 -> Logger/109
  Constant9/1 -> Logger/110
  Constant10/1 -> Logger/111
  Constant11/1 -> Logger/112
  Constant12/1 -> Logger/113
  Constant13/1 -> Logger/114
  Constant14/1 -> Logger/115
  Constant15/1 -> Logger/116
  [sigEngine] -> Bus Selector2/1
  Bus Selector2/1 -> Logger/117  "<engineN>"
  [sigGearbox] -> Bus Selector3/1
  Bus Selector3/1 -> Logger/118  "<gearPosView>"
  [sigChassis] -> Bus Selector4/1
  Bus Selector4/1 -> vectorLength/1  "<localVel>"
  vectorLength/1 -> Logger/119
  Bus Selector4/4 -> Logger/126  "<odo>"
  Demux1/1 -> Logger/120
  Demux1/2 -> Logger/121
  Demux1/3 -> Logger/122
  Demux/1 -> Logger/123
  Demux/2 -> Logger/124
  Demux/3 -> Logger/125
  Bus Selector4/3 -> Demux/1  "<posCG>"
  Bus Selector4/2 -> Demux1/1  "<localAccNoRollPitch>"
  [sigEngine] -> Bus Selector5/1
  Bus Selector5/1 -> Logger/142  "<throttle>"
  [sigBrake] -> Bus Selector6/1
  Bus Selector6/1 -> Logger/143  "<brakeFront>"
  [sigClutch] -> Bus Selector7/1
  Bus Selector7/1 -> Logger/144  "<clutch>"
  Constant20/1 -> Logger/141
  Constant19/1 -> Logger/140
  Constant18/1 -> Logger/139
  Constant31/1 -> Logger/138
  Constant30/1 -> Logger/137
  Constant29/1 -> Logger/136
  Constant28/1 -> Logger/135
  Constant27/1 -> Logger/134
  Constant26/1 -> Logger/133
  Constant25/1 -> Logger/132
  Constant24/1 -> Logger/131
  Constant17/1 -> Logger/130
  loggerInfo/1 -> Bus Selector/1
  Bus Selector/1 -> Logger/127  "<distance>"
  Bus Selector/2 -> Logger/128  "<lapCount>"
  Bus Selector/3 -> Logger/129  "<sectorCount>"
  Bus Selector31/1 -> Logger/65  "<rho>"
  Bus Selector31/2 -> Logger/66  "<rho>"
  Bus Selector31/3 -> Logger/67  "<rho>"
  Bus Selector31/4 -> Logger/68  "<rho>"
  Bus Selector31/9 -> Logger/77  "<kappa>"
  Bus Selector31/10 -> Logger/78  "<kappa>"
  Bus Selector31/11 -> Logger/79  "<kappa>"
  Bus Selector31/12 -> Logger/80  "<kappa>"
  Bus Selector31/13 -> rad to deg33/1  "<alpha>"
  Bus Selector31/14 -> rad to deg34/1  "<alpha>"
  Bus Selector31/15 -> rad to deg35/1  "<alpha>"
  Bus Selector31/16 -> rad to deg36/1  "<alpha>"
  Bus Selector31/20 -> Logger/88  "<FxC>"
  Bus Selector31/19 -> Logger/87  "<FxC>"
  Bus Selector31/18 -> Logger/86  "<FxC>"
  Bus Selector31/17 -> Logger/85  "<FxC>"
  Constant32/1 -> Logger/7
  Constant33/1 -> Logger/24
  Constant34/1 -> Logger/25
  Constant35/1 -> Logger/26
  Constant36/1 -> Logger/27
  Constant37/1 -> Logger/28
  Constant38/1 -> Logger/29
